simulink model "vctrlsystem"  (R2022b)
settings: Solver=VariableStepAuto  StartTime=0.0  StopTime=3  RelTol=1e-3
undefined symbols (not defined in the file): K, Kp, sigma
libraries: simulink x1
settings Model: Creator=JackPaul  LastModifiedBy=JackPaul

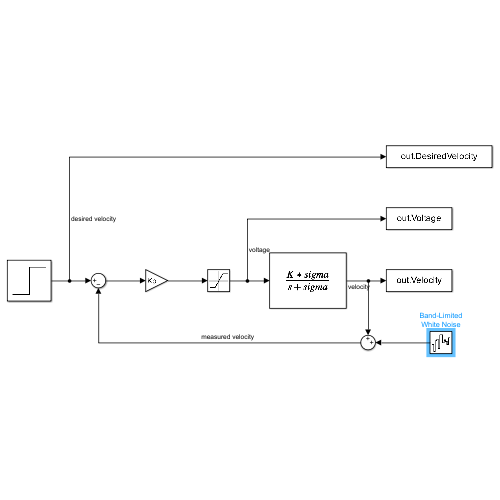
[thumbnail: Simulink's stored preview of the top-level diagram]
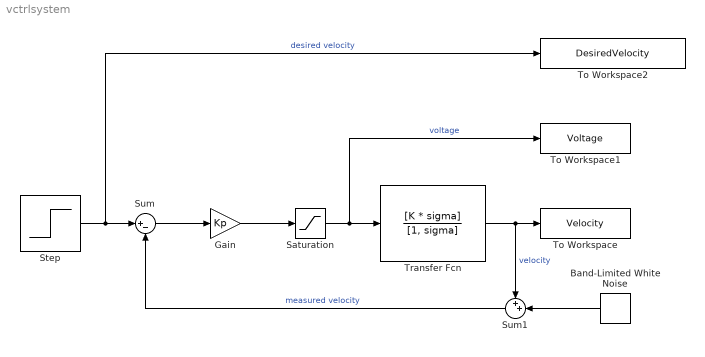
== system vctrlsystem ==
  Band-Limited White Noise : simulink/Sources/Band-Limited White Noise  Cov=[0.0001]  Ts=0.01  seed=[444444]
  Gain : Gain  Gain=Kp
  Saturation : Saturate  UpperLimit=7.5  LowerLimit=-7.5
  Step : Step  SampleTime=0
  Sum : Sum  Inputs=|+-
  Sum1 : Sum  Inputs=++|
  To Workspace : ToWorkspace  VariableName=Velocity  SaveFormat=Timeseries  SampleTime=-1
  To Workspace1 : ToWorkspace  VariableName=Voltage  SaveFormat=Timeseries  SampleTime=-1
  To Workspace2 : ToWorkspace  VariableName=DesiredVelocity  SaveFormat=Timeseries  SampleTime=-1
  Transfer Fcn : TransferFcn  Numerator=[K * sigma]  Denominator=[1, sigma]  ParameterTunability=Unconstrained
  wires:
  Band-Limited White Noise/1 -> Sum1/2
  Transfer Fcn/1 -> Sum1/1, To Workspace/1  "velocity"
  Saturation/1 -> To Workspace1/1, Transfer Fcn/1  "voltage"
  Gain/1 -> Saturation/1
  Sum/1 -> Gain/1
  Step/1 -> To Workspace2/1, Sum/1  "desired velocity"
  Sum1/1 -> Sum/2  "measured velocity"
